simulink model "LAB11_sim_1"  (R2022b)
settings: Solver=VariableStepAuto  StartTime=0.0  StopTime=czas_symulacji  MaxStep=0.1  RelTol=1e-3
values from neighbouring files (symbols this model uses):
  Cvp = cp*rop*Vp    (= 14400)    [LAB11_1.m]
  Cvw = cp*rop*Vw    (= 96000)    [LAB11_1.m]
  drugi_step_time = 3000    [LAB11_1.m]
  dTp = 2    [LAB11_1.m]
  dTp2 = 10    [LAB11_1.m]
  dTzew = 0    [LAB11_1.m]
  Kb = 500    [LAB11_1.m]
  Kcp = (a*QgN)*(TwewN-TpN)/((TpN-TzewN)*(TwewN-TzewN+a*(TwewN-TpN)))    (= 23.2558139535)    [LAB11_1.m]
  Kcw = (QgN)/(TwewN-TzewN+a*TwewN-a*TpN)    (= 232.558139535)    [LAB11_1.m]
  Kcwp = (a*QgN)/(TwewN-TzewN+a*TwewN-a*TpN)    (= 69.7674418605)    [LAB11_1.m]
  lower_limit = 0    [LAB11_1.m]
  spadekTp = -10    [LAB11_1.m]
  t0 = 1000    [LAB11_1.m]
  Tp0 = (Kcp*Tzew0*(Kcw+Kcwp)+Kcwp*(Qg0+Kcw*Tzew0))/(Kcw*Kcwp+Kcw*Kcp+Kcwp*Kcp)    (= 17)    [LAB11_1.m]
  Twew0 = (Qg0+Kcw*Tzew0+a*Kcw*Tp0)/(Kcw+Kcwp)    (= 27)    [LAB11_1.m]
  Tzew0 = TzewN+7    (= -13)    [LAB11_1.m]
  upper_limit = 11500    [LAB11_1.m]
libraries: slpidlib x6
settings Model: Creator=maciejrudy  LastModifiedBy=Dawkin
settings SolverCC: AlgebraicLoopSolver=TrustRegion
settings DataIOCC: ReturnWorkspaceOutputs=off
settings DebuggingCC: UnconnectedInputMsg=warning  UnconnectedOutputMsg=warning  UnconnectedLineMsg=warning  SFMachineParentedDataDiag=warning
settings ModelReferenceCC: EnableRefExpFcnMdlSchedulingChecks=on
settings RTWCC: DLArmComputeVersion=19.05

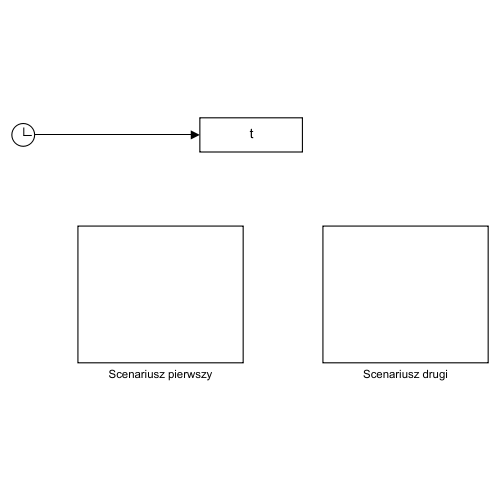
[thumbnail: Simulink's stored preview of the top-level diagram]
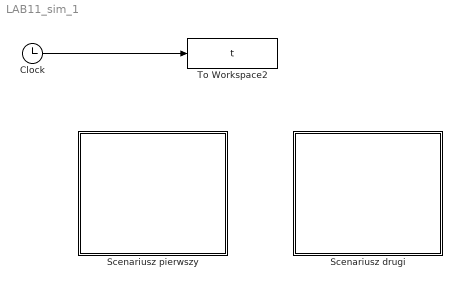
== system LAB11_sim_1 ==
  Clock : Clock
  Scenariusz drugi : Subsystem
  Scenariusz pierwszy : Subsystem
  To Workspace2 : ToWorkspace  VariableName=t  SaveFormat=Timeseries  SampleTime=-1
  wires:
  Clock/1 -> To Workspace2/1

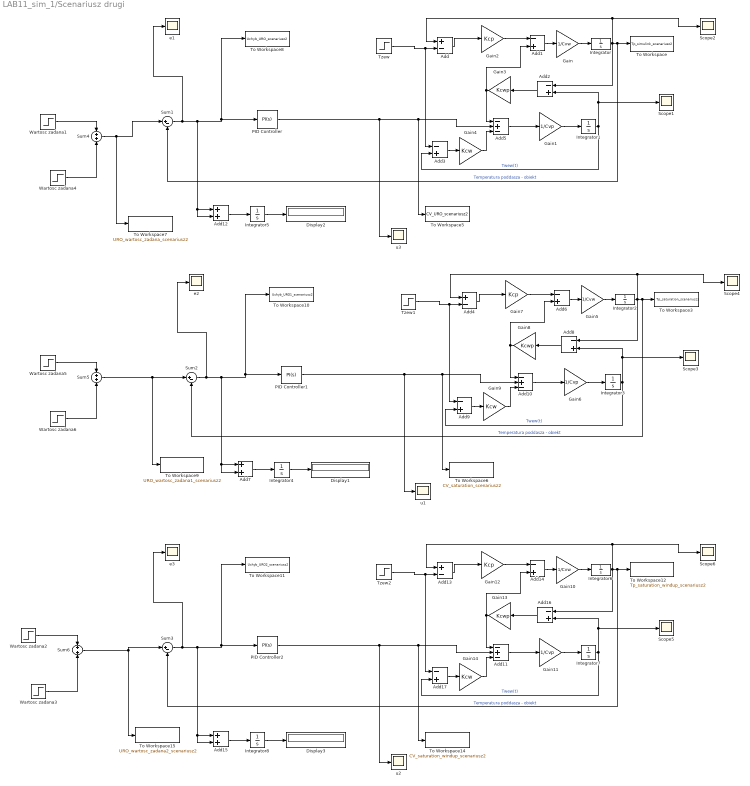
== system LAB11_sim_1/Scenariusz drugi ==
  Add : Sum  Inputs=+-
  Add{1..3,6,8..9,14,16..17} (9 alike) : Sum  Inputs=-+
  Add10 : Sum  Inputs=-+-
  Add11 : Sum  Inputs=-+-
  Add12 : Sum
  Add13 : Sum  Inputs=+-
  Add15 : Sum
  Add4 : Sum  Inputs=+-
  Add5 : Sum  Inputs=-+-
  Add7 : Sum
  Display1 : Display
  Display2 : Display
  Display3 : Display
  Gain : Gain  Gain=1/Cvw
  Gain1 : Gain  Gain=1/Cvp
  Gain10 : Gain  Gain=1/Cvw
  Gain11 : Gain  Gain=1/Cvp
  Gain12 : Gain  Gain=Kcp
  Gain13 : Gain  Gain=Kcwp
  Gain14 : Gain  Gain=Kcw
  Gain2 : Gain  Gain=Kcp
  Gain3 : Gain  Gain=Kcwp
  Gain4 : Gain  Gain=Kcw
  Gain5 : Gain  Gain=1/Cvw
  Gain6 : Gain  Gain=1/Cvp
  Gain7 : Gain  Gain=Kcp
  Gain8 : Gain  Gain=Kcwp
  Gain9 : Gain  Gain=Kcw
  Integrator : Integrator  InitialCondition=Tp0
  Integrator1 : Integrator  InitialCondition=Twew0
  Integrator2 : Integrator  InitialCondition=Tp0
  Integrator3 : Integrator  InitialCondition=Twew0
  Integrator4 : Integrator
  Integrator5 : Integrator
  Integrator6 : Integrator  InitialCondition=Tp0
  Integrator7 : Integrator  InitialCondition=Twew0
  Integrator8 : Integrator
  PID Controller : slpidlib/PID Controller  Controller=PI  Form=Parallel  TimeDomain=Continuous-time  UseExternalTs=off  SampleTime=-1  IntegratorMethod=Forward Euler  FilterMethod=Forward Euler  ControllerParametersSource=internal  P=2386.66771221404  I=38.2166019284268  UseKiTs=off  D=0  N=100  UseFilter=on  TunerSelectOption=Transfer Function Based (PID Tuner App)  InitialConditionSource=internal  InitialConditionForIntegrator=Qg0  InitialConditionForFilter=0  DifferentiatorICPrevScaledInput=0  ExternalReset=none  TrackingMode=off  Kt=1  LimitOutput=off  SatLimitsSource=internal  UpperSaturationLimit=upper_limit  LowerSaturationLimit=lower_limit  LinearizeAsGain=on  AntiWindupMode=back-calculation  Kb=Kb  LimitIntegrator=off  UpperIntegratorSaturationLimit=inf  LowerIntegratorSaturationLimit=-inf  POutMin=[]  POutMax=[]  IOutMin=[]  IOutMax=[]  DOutMin=[]  DOutMax=[]  NOutMin=[]  NOutMax=[]  SumOutMin=[]  SumOutMax=[]  SaturationOutMin=[]  SaturationOutMax=[]  PParamMin=[]  PParamMax=[]  IParamMin=[]  IParamMax=[]  DParamMin=[]  DParamMax=[]  NParamMin=[]  NParamMax=[]  KbParamMin=[]  KbParamMax=[]  KtParamMin=[]  KtParamMax=[]  KbOutMin=[]  KbOutMax=[]  KtOutMin=[]  KtOutMax=[]  IntegratorOutMin=[]  IntegratorOutMax=[]  FilterOutMin=[]  FilterOutMax=[]  SumI1OutMin=[]  SumI1OutMax=[]  SumI2OutMin=[]  SumI2OutMax=[]  SumI3OutMin=[]  SumI3OutMax=[]  SumI4OutMin=[]  SumI4OutMax=[]  SumDOutMin=[]  SumDOutMax=[]  DifferentiatorOutMin=[]  DifferentiatorOutMax=[]  FilterDiffOutCoefMin=[]  FilterDiffOutCoefMax=[]  ReciprocalOutMin=[]  ReciprocalOutMax=[]  SumDenOutMin=[]  SumDenOutMax=[]  SumNumOutMin=[]  SumNumOutMax=[]  DivideOutMin=[]  DivideOutMax=[]  UdiffTsProdOutMin=[]  UdiffTsProdOutMax=[]  NTsProdOutMin=[]  NTsProdOutMax=[]  UintegralTsProdOutMin=[]  UintegralTsProdOutMax=[]  UngainTsProdOutMin=[]  UngainTsProdOutMax=[]  ClampingZeroOutDataTypeStr=Inherit: Inherit via back propagation  ClampingZeroOutMin=[]  ClampingZeroOutMax=[]  FilterDenConstantOutDataTypeStr=Inherit: Inherit via back propagation  FilterDenConstantOutMin=[]  FilterDenConstantOutMax=[]  PCopyOutDataTypeStr=Inherit: Inherit via back propagation  PCopyOutMin=[]  PCopyOutMax=[]  NCopyOutDataTypeStr=Inherit: Inherit via back propagation  NCopyOutMin=[]  NCopyOutMax=[]  IntegratorContinuousStateAttributes=''  IntegratorStateMustResolveToSignalObject=off  IntegratorRTWStateStorageClass=Auto  FilterContinuousStateAttributes=''  FilterStateMustResolveToSignalObject=off  FilterRTWStateStorageClass=Auto  ParallelPVariant=InternalParameters  IdealPVariant=Disabled  IVariant=InternalParameters  DVariant=Disabled  IntegratorVariant=Continuous  SatVariant=Disabled  AWVariant=Passthrough  PCopyVariant=Disabled  TRVariant=Disabled  FdbkBlocksVariant=Forward  IdealPFdbkVariant=Disabled  SatFdbkVariant=Disabled  DerivativeFilterVariant=Disabled  NVariant=Disabled  NCopyVariant=Disabled_SignalSpec  FilterICVariant=Disabled  IntegratorICVariant=InternalICs  ExternalResetVariant=Disabled  TRSumVariant=Passthrough  SumFdbkVariant=Disabled  SumVariant=Sum_PI  TsampFilterVariant=InternalTs  TsampNgainVariant=Passthrough  TsampIntegralVariant=Passthrough  ExternalSaturationOutDataTypeStr=Inherit: Same as second input
  PID Controller1 : slpidlib/PID Controller  Controller=PI  Form=Parallel  TimeDomain=Continuous-time  UseExternalTs=off  SampleTime=-1  IntegratorMethod=Forward Euler  FilterMethod=Forward Euler  ControllerParametersSource=internal  P=2386.66771221404  I=38.2166019284268  UseKiTs=off  D=0  N=100  UseFilter=on  TunerSelectOption=Transfer Function Based (PID Tuner App)  InitialConditionSource=internal  InitialConditionForIntegrator=Qg0  InitialConditionForFilter=0  DifferentiatorICPrevScaledInput=0  ExternalReset=none  TrackingMode=off  Kt=1  LimitOutput=on  SatLimitsSource=internal  UpperSaturationLimit=upper_limit  LowerSaturationLimit=lower_limit  LinearizeAsGain=on  AntiWindupMode=none  Kb=Kb  LimitIntegrator=off  UpperIntegratorSaturationLimit=inf  LowerIntegratorSaturationLimit=-inf  POutMin=[]  POutMax=[]  IOutMin=[]  IOutMax=[]  DOutMin=[]  DOutMax=[]  NOutMin=[]  NOutMax=[]  SumOutMin=[]  SumOutMax=[]  SaturationOutMin=[]  SaturationOutMax=[]  PParamMin=[]  PParamMax=[]  IParamMin=[]  IParamMax=[]  DParamMin=[]  DParamMax=[]  NParamMin=[]  NParamMax=[]  KbParamMin=[]  KbParamMax=[]  KtParamMin=[]  KtParamMax=[]  KbOutMin=[]  KbOutMax=[]  KtOutMin=[]  KtOutMax=[]  IntegratorOutMin=[]  IntegratorOutMax=[]  FilterOutMin=[]  FilterOutMax=[]  SumI1OutMin=[]  SumI1OutMax=[]  SumI2OutMin=[]  SumI2OutMax=[]  SumI3OutMin=[]  SumI3OutMax=[]  SumI4OutMin=[]  SumI4OutMax=[]  SumDOutMin=[]  SumDOutMax=[]  DifferentiatorOutMin=[]  DifferentiatorOutMax=[]  FilterDiffOutCoefMin=[]  FilterDiffOutCoefMax=[]  ReciprocalOutMin=[]  ReciprocalOutMax=[]  SumDenOutMin=[]  SumDenOutMax=[]  SumNumOutMin=[]  SumNumOutMax=[]  DivideOutMin=[]  DivideOutMax=[]  UdiffTsProdOutMin=[]  UdiffTsProdOutMax=[]  NTsProdOutMin=[]  NTsProdOutMax=[]  UintegralTsProdOutMin=[]  UintegralTsProdOutMax=[]  UngainTsProdOutMin=[]  UngainTsProdOutMax=[]  ClampingZeroOutDataTypeStr=Inherit: Inherit via back propagation  ClampingZeroOutMin=[]  ClampingZeroOutMax=[]  FilterDenConstantOutDataTypeStr=Inherit: Inherit via back propagation  FilterDenConstantOutMin=[]  FilterDenConstantOutMax=[]  PCopyOutDataTypeStr=Inherit: Inherit via back propagation  PCopyOutMin=[]  PCopyOutMax=[]  NCopyOutDataTypeStr=Inherit: Inherit via back propagation  NCopyOutMin=[]  NCopyOutMax=[]  IntegratorContinuousStateAttributes=''  IntegratorStateMustResolveToSignalObject=off  IntegratorRTWStateStorageClass=Auto  FilterContinuousStateAttributes=''  FilterStateMustResolveToSignalObject=off  FilterRTWStateStorageClass=Auto  ParallelPVariant=InternalParameters  IdealPVariant=Disabled  IVariant=InternalParameters  DVariant=Disabled  IntegratorVariant=Continuous  SatVariant=Enabled  AWVariant=Passthrough  PCopyVariant=Disabled  TRVariant=Disabled  FdbkBlocksVariant=Forward  IdealPFdbkVariant=Disabled  SatFdbkVariant=Disabled  DerivativeFilterVariant=Disabled  NVariant=Disabled  NCopyVariant=Disabled_SignalSpec  FilterICVariant=Disabled  IntegratorICVariant=InternalICs  ExternalResetVariant=Disabled  TRSumVariant=Passthrough  SumFdbkVariant=Disabled  SumVariant=Sum_PI  TsampFilterVariant=InternalTs  TsampNgainVariant=Passthrough  TsampIntegralVariant=Passthrough  ExternalSaturationOutDataTypeStr=Inherit: Same as second input
  PID Controller2 : slpidlib/PID Controller  Controller=PI  Form=Parallel  TimeDomain=Continuous-time  UseExternalTs=off  SampleTime=-1  IntegratorMethod=Forward Euler  FilterMethod=Forward Euler  ControllerParametersSource=internal  P=2386.66771221404  I=38.2166019284268  UseKiTs=off  D=0  N=100  UseFilter=on  TunerSelectOption=Transfer Function Based (PID Tuner App)  InitialConditionSource=internal  InitialConditionForIntegrator=Qg0  InitialConditionForFilter=0  DifferentiatorICPrevScaledInput=0  ExternalReset=none  TrackingMode=off  Kt=1  LimitOutput=on  SatLimitsSource=internal  UpperSaturationLimit=upper_limit  LowerSaturationLimit=lower_limit  LinearizeAsGain=on  AntiWindupMode=back-calculation  Kb=Kb  LimitIntegrator=off  UpperIntegratorSaturationLimit=inf  LowerIntegratorSaturationLimit=-inf  POutMin=[]  POutMax=[]  IOutMin=[]  IOutMax=[]  DOutMin=[]  DOutMax=[]  NOutMin=[]  NOutMax=[]  SumOutMin=[]  SumOutMax=[]  SaturationOutMin=[]  SaturationOutMax=[]  PParamMin=[]  PParamMax=[]  IParamMin=[]  IParamMax=[]  DParamMin=[]  DParamMax=[]  NParamMin=[]  NParamMax=[]  KbParamMin=[]  KbParamMax=[]  KtParamMin=[]  KtParamMax=[]  KbOutMin=[]  KbOutMax=[]  KtOutMin=[]  KtOutMax=[]  IntegratorOutMin=[]  IntegratorOutMax=[]  FilterOutMin=[]  FilterOutMax=[]  SumI1OutMin=[]  SumI1OutMax=[]  SumI2OutMin=[]  SumI2OutMax=[]  SumI3OutMin=[]  SumI3OutMax=[]  SumI4OutMin=[]  SumI4OutMax=[]  SumDOutMin=[]  SumDOutMax=[]  DifferentiatorOutMin=[]  DifferentiatorOutMax=[]  FilterDiffOutCoefMin=[]  FilterDiffOutCoefMax=[]  ReciprocalOutMin=[]  ReciprocalOutMax=[]  SumDenOutMin=[]  SumDenOutMax=[]  SumNumOutMin=[]  SumNumOutMax=[]  DivideOutMin=[]  DivideOutMax=[]  UdiffTsProdOutMin=[]  UdiffTsProdOutMax=[]  NTsProdOutMin=[]  NTsProdOutMax=[]  UintegralTsProdOutMin=[]  UintegralTsProdOutMax=[]  UngainTsProdOutMin=[]  UngainTsProdOutMax=[]  ClampingZeroOutDataTypeStr=Inherit: Inherit via back propagation  ClampingZeroOutMin=[]  ClampingZeroOutMax=[]  FilterDenConstantOutDataTypeStr=Inherit: Inherit via back propagation  FilterDenConstantOutMin=[]  FilterDenConstantOutMax=[]  PCopyOutDataTypeStr=Inherit: Inherit via back propagation  PCopyOutMin=[]  PCopyOutMax=[]  NCopyOutDataTypeStr=Inherit: Inherit via back propagation  NCopyOutMin=[]  NCopyOutMax=[]  IntegratorContinuousStateAttributes=''  IntegratorStateMustResolveToSignalObject=off  IntegratorRTWStateStorageClass=Auto  FilterContinuousStateAttributes=''  FilterStateMustResolveToSignalObject=off  FilterRTWStateStorageClass=Auto  ParallelPVariant=InternalParameters  IdealPVariant=Disabled  IVariant=InternalParameters  DVariant=Disabled  IntegratorVariant=Continuous  SatVariant=Enabled  AWVariant=BackCalculation  PCopyVariant=Disabled  TRVariant=Disabled  FdbkBlocksVariant=Forward  IdealPFdbkVariant=Disabled  SatFdbkVariant=Disabled  DerivativeFilterVariant=Disabled  NVariant=Disabled  NCopyVariant=Disabled_SignalSpec  FilterICVariant=Disabled  IntegratorICVariant=InternalICs  ExternalResetVariant=Disabled  TRSumVariant=Passthrough  SumFdbkVariant=Disabled  SumVariant=Sum_PI  TsampFilterVariant=InternalTs  TsampNgainVariant=Passthrough  TsampIntegralVariant=Passthrough  ExternalSaturationOutDataTypeStr=Inherit: Same as second input
  Scope{1..6} (6 alike) : Scope
  Sum1 : Sum  Inputs=|+-
  Sum2 : Sum  Inputs=|+-
  Sum3 : Sum  Inputs=|+-
  Sum4 : Sum
  Sum5 : Sum
  Sum6 : Sum
  To Workspace : ToWorkspace  VariableName=Tp_simulink_scenariusz2  SampleTime=-1
  To Workspace10 : ToWorkspace  VariableName=Uchyb_URO1_scenariusz2  SampleTime=-1
  To Workspace11 : ToWorkspace  VariableName=Uchyb_URO2_scenariusz2  SampleTime=-1
  To Workspace12 : ToWorkspace  VariableName=Tp_saturation_windup_scenariusz2  SampleTime=-1
  To Workspace14 : ToWorkspace  VariableName=CV_saturation_windup_scenariusz2  SampleTime=-1
  To Workspace15 : ToWorkspace  VariableName=URO_wartosc_zadana2_scenariusz2  SampleTime=-1
  To Workspace3 : ToWorkspace  VariableName=Tp_saturation_scenariusz2  SampleTime=-1
  To Workspace5 : ToWorkspace  VariableName=CV_URO_scenariusz2  SampleTime=-1
  To Workspace6 : ToWorkspace  VariableName=CV_saturation_scenariusz2  SampleTime=-1
  To Workspace7 : ToWorkspace  VariableName=URO_wartosc_zadana_scenariusz2  SampleTime=-1
  To Workspace8 : ToWorkspace  VariableName=Uchyb_URO_scenariusz2  SampleTime=-1
  To Workspace9 : ToWorkspace  VariableName=URO_wartosc_zadana1_scenariusz2  SampleTime=-1
  Tzew : Step  Time=t0  Before=Tzew0  After=Tzew0+dTzew  SampleTime=0
  Tzew1 : Step  Time=t0  Before=Tzew0  After=Tzew0+dTzew  SampleTime=0
  Tzew2 : Step  Time=t0  Before=Tzew0  After=Tzew0+dTzew  SampleTime=0
  Wartosc zadana1 : Step  Time=t0  Before=Tp0  After=Tp0+dTp2  SampleTime=0
  Wartosc zadana2 : Step  Time=t0  Before=Tp0  After=Tp0+dTp2  SampleTime=0
  Wartosc zadana3 : Step  Time=drugi_step_time  After=spadekTp  SampleTime=0
  Wartosc zadana4 : Step  Time=drugi_step_time  After=spadekTp  SampleTime=0
  Wartosc zadana5 : Step  Time=t0  Before=Tp0  After=Tp0+dTp2  SampleTime=0
  Wartosc zadana6 : Step  Time=drugi_step_time  After=spadekTp  SampleTime=0
  e1 : Scope
  e2 : Scope
  e3 : Scope
  u1 : Scope
  u2 : Scope
  u3 : Scope
  wires:
  Gain12/1 -> Add14/1
  Gain11/1 -> Integrator7/1
  Integrator6/1 -> Add16/1, To Workspace12/1, Sum3/2, Scope6/1, Add13/1  "Temperatura poddasza - obiekt"
  Add17/1 -> Gain14/1
  Gain4/1 -> Add5/3
  Add5/1 -> Gain1/1
  Gain14/1 -> Add11/3
  Gain/1 -> Integrator/1
  Tzew2/1 -> Add17/1, Add13/2
  Add/1 -> Gain2/1
  Add15/1 -> Integrator8/1
  Add8/1 -> Gain8/1
  Add10/1 -> Gain6/1
  PID Controller/1 -> To Workspace5/1, Add5/2, u3/1
  Add12/1 -> Integrator5/1
  Gain6/1 -> Integrator3/1
  Add7/1 -> Integrator4/1
  Add2/1 -> Gain3/1
  Gain3/1 -> Add5/1, Add1/2
  Add9/1 -> Gain9/1
  PID Controller2/1 -> To Workspace14/1, Add11/2, u2/1
  Add11/1 -> Gain11/1
  Gain13/1 -> Add11/1, Add14/2
  Tzew/1 -> Add3/1, Add/2
  Integrator8/1 -> Display3/1
  Gain1/1 -> Integrator1/1
  Add16/1 -> Gain13/1
  Integrator7/1 -> Add17/2, Add16/2, Scope5/1  "Twew(t)"
  Add13/1 -> Gain12/1
  Integrator/1 -> Add2/1, To Workspace/1, Sum1/2, Scope2/1, Add/1  "Temperatura poddasza - obiekt"
  Gain9/1 -> Add10/3
  Integrator5/1 -> Display2/1
  Sum6/1 -> Sum3/1, To Workspace15/1
  Gain5/1 -> Integrator2/1
  Tzew1/1 -> Add9/1, Add4/2
  Add14/1 -> Gain10/1
  Integrator4/1 -> Display1/1
  Sum5/1 -> To Workspace9/1, Sum2/1
  Integrator3/1 -> Add9/2, Add8/2, Scope3/1  "Twew(t)"
  Add6/1 -> Gain5/1
  Add3/1 -> Gain4/1
  Gain2/1 -> Add1/1
  Add1/1 -> Gain/1
  Sum2/1 -> e2/1, PID Controller1/1, To Workspace10/1, Add7/2, Add7/1
  PID Controller1/1 -> To Workspace6/1, Add10/2, u1/1
  Sum1/1 -> e1/1, PID Controller/1, To Workspace8/1, Add12/2, Add12/1
  Gain7/1 -> Add6/1
  Gain8/1 -> Add10/1, Add6/2
  Integrator1/1 -> Add3/2, Add2/2, Scope1/1  "Twew(t)"
  Sum3/1 -> e3/1, PID Controller2/1, To Workspace11/1, Add15/2, Add15/1
  Gain10/1 -> Integrator6/1
  Integrator2/1 -> Add8/1, To Workspace3/1, Sum2/2, Scope4/1, Add4/1  "Temperatura poddasza - obiekt"
  Add4/1 -> Gain7/1
  Wartosc zadana4/1 -> Sum4/2
  Wartosc zadana1/1 -> Sum4/1
  Sum4/1 -> Sum1/1, To Workspace7/1
  Wartosc zadana6/1 -> Sum5/2
  Wartosc zadana5/1 -> Sum5/1
  Wartosc zadana3/1 -> Sum6/2
  Wartosc zadana2/1 -> Sum6/1

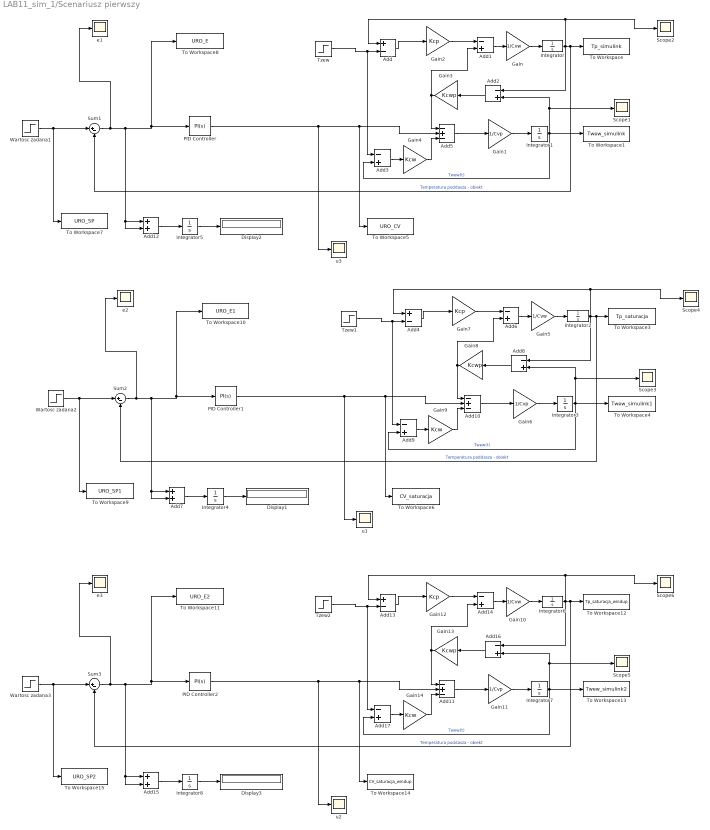
== system LAB11_sim_1/Scenariusz pierwszy ==
  Add : Sum  Inputs=+-
  Add{1..3,6,8..9,14,16..17} (9 alike) : Sum  Inputs=-+
  Add10 : Sum  Inputs=-+-
  Add11 : Sum  Inputs=-+-
  Add12 : Sum
  Add13 : Sum  Inputs=+-
  Add15 : Sum
  Add4 : Sum  Inputs=+-
  Add5 : Sum  Inputs=-+-
  Add7 : Sum
  Display1 : Display
  Display2 : Display
  Display3 : Display
  Gain : Gain  Gain=1/Cvw
  Gain1 : Gain  Gain=1/Cvp
  Gain10 : Gain  Gain=1/Cvw
  Gain11 : Gain  Gain=1/Cvp
  Gain12 : Gain  Gain=Kcp
  Gain13 : Gain  Gain=Kcwp
  Gain14 : Gain  Gain=Kcw
  Gain2 : Gain  Gain=Kcp
  Gain3 : Gain  Gain=Kcwp
  Gain4 : Gain  Gain=Kcw
  Gain5 : Gain  Gain=1/Cvw
  Gain6 : Gain  Gain=1/Cvp
  Gain7 : Gain  Gain=Kcp
  Gain8 : Gain  Gain=Kcwp
  Gain9 : Gain  Gain=Kcw
  Integrator : Integrator  InitialCondition=Tp0
  Integrator1 : Integrator  InitialCondition=Twew0
  Integrator2 : Integrator  InitialCondition=Tp0
  Integrator3 : Integrator  InitialCondition=Twew0
  Integrator4 : Integrator
  Integrator5 : Integrator
  Integrator6 : Integrator  InitialCondition=Tp0
  Integrator7 : Integrator  InitialCondition=Twew0
  Integrator8 : Integrator
  PID Controller : slpidlib/PID Controller  Controller=PI  Form=Parallel  TimeDomain=Continuous-time  UseExternalTs=off  SampleTime=-1  IntegratorMethod=Forward Euler  FilterMethod=Forward Euler  ControllerParametersSource=internal  P=2386.66771221404  I=38.2166019284268  UseKiTs=off  D=0  N=100  UseFilter=on  TunerSelectOption=Transfer Function Based (PID Tuner App)  InitialConditionSource=internal  InitialConditionForIntegrator=Qg0  InitialConditionForFilter=0  DifferentiatorICPrevScaledInput=0  ExternalReset=none  TrackingMode=off  Kt=1  LimitOutput=off  SatLimitsSource=internal  UpperSaturationLimit=upper_limit  LowerSaturationLimit=lower_limit  LinearizeAsGain=on  AntiWindupMode=back-calculation  Kb=Kb  LimitIntegrator=off  UpperIntegratorSaturationLimit=inf  LowerIntegratorSaturationLimit=-inf  POutMin=[]  POutMax=[]  IOutMin=[]  IOutMax=[]  DOutMin=[]  DOutMax=[]  NOutMin=[]  NOutMax=[]  SumOutMin=[]  SumOutMax=[]  SaturationOutMin=[]  SaturationOutMax=[]  PParamMin=[]  PParamMax=[]  IParamMin=[]  IParamMax=[]  DParamMin=[]  DParamMax=[]  NParamMin=[]  NParamMax=[]  KbParamMin=[]  KbParamMax=[]  KtParamMin=[]  KtParamMax=[]  KbOutMin=[]  KbOutMax=[]  KtOutMin=[]  KtOutMax=[]  IntegratorOutMin=[]  IntegratorOutMax=[]  FilterOutMin=[]  FilterOutMax=[]  SumI1OutMin=[]  SumI1OutMax=[]  SumI2OutMin=[]  SumI2OutMax=[]  SumI3OutMin=[]  SumI3OutMax=[]  SumI4OutMin=[]  SumI4OutMax=[]  SumDOutMin=[]  SumDOutMax=[]  DifferentiatorOutMin=[]  DifferentiatorOutMax=[]  FilterDiffOutCoefMin=[]  FilterDiffOutCoefMax=[]  ReciprocalOutMin=[]  ReciprocalOutMax=[]  SumDenOutMin=[]  SumDenOutMax=[]  SumNumOutMin=[]  SumNumOutMax=[]  DivideOutMin=[]  DivideOutMax=[]  UdiffTsProdOutMin=[]  UdiffTsProdOutMax=[]  NTsProdOutMin=[]  NTsProdOutMax=[]  UintegralTsProdOutMin=[]  UintegralTsProdOutMax=[]  UngainTsProdOutMin=[]  UngainTsProdOutMax=[]  ClampingZeroOutDataTypeStr=Inherit: Inherit via back propagation  ClampingZeroOutMin=[]  ClampingZeroOutMax=[]  FilterDenConstantOutDataTypeStr=Inherit: Inherit via back propagation  FilterDenConstantOutMin=[]  FilterDenConstantOutMax=[]  PCopyOutDataTypeStr=Inherit: Inherit via back propagation  PCopyOutMin=[]  PCopyOutMax=[]  NCopyOutDataTypeStr=Inherit: Inherit via back propagation  NCopyOutMin=[]  NCopyOutMax=[]  IntegratorContinuousStateAttributes=''  IntegratorStateMustResolveToSignalObject=off  IntegratorRTWStateStorageClass=Auto  FilterContinuousStateAttributes=''  FilterStateMustResolveToSignalObject=off  FilterRTWStateStorageClass=Auto  ParallelPVariant=InternalParameters  IdealPVariant=Disabled  IVariant=InternalParameters  DVariant=Disabled  IntegratorVariant=Continuous  SatVariant=Disabled  AWVariant=Passthrough  PCopyVariant=Disabled  TRVariant=Disabled  FdbkBlocksVariant=Forward  IdealPFdbkVariant=Disabled  SatFdbkVariant=Disabled  DerivativeFilterVariant=Disabled  NVariant=Disabled  NCopyVariant=Disabled_SignalSpec  FilterICVariant=Disabled  IntegratorICVariant=InternalICs  ExternalResetVariant=Disabled  TRSumVariant=Passthrough  SumFdbkVariant=Disabled  SumVariant=Sum_PI  TsampFilterVariant=InternalTs  TsampNgainVariant=Passthrough  TsampIntegralVariant=Passthrough  ExternalSaturationOutDataTypeStr=Inherit: Same as second input
  PID Controller1 : slpidlib/PID Controller  Controller=PI  Form=Parallel  TimeDomain=Continuous-time  UseExternalTs=off  SampleTime=-1  IntegratorMethod=Forward Euler  FilterMethod=Forward Euler  ControllerParametersSource=internal  P=2386.66771221404  I=38.2166019284268  UseKiTs=off  D=0  N=100  UseFilter=on  TunerSelectOption=Transfer Function Based (PID Tuner App)  InitialConditionSource=internal  InitialConditionForIntegrator=Qg0  InitialConditionForFilter=0  DifferentiatorICPrevScaledInput=0  ExternalReset=none  TrackingMode=off  Kt=1  LimitOutput=on  SatLimitsSource=internal  UpperSaturationLimit=upper_limit  LowerSaturationLimit=lower_limit  LinearizeAsGain=on  AntiWindupMode=none  Kb=Kb  LimitIntegrator=off  UpperIntegratorSaturationLimit=inf  LowerIntegratorSaturationLimit=-inf  POutMin=[]  POutMax=[]  IOutMin=[]  IOutMax=[]  DOutMin=[]  DOutMax=[]  NOutMin=[]  NOutMax=[]  SumOutMin=[]  SumOutMax=[]  SaturationOutMin=[]  SaturationOutMax=[]  PParamMin=[]  PParamMax=[]  IParamMin=[]  IParamMax=[]  DParamMin=[]  DParamMax=[]  NParamMin=[]  NParamMax=[]  KbParamMin=[]  KbParamMax=[]  KtParamMin=[]  KtParamMax=[]  KbOutMin=[]  KbOutMax=[]  KtOutMin=[]  KtOutMax=[]  IntegratorOutMin=[]  IntegratorOutMax=[]  FilterOutMin=[]  FilterOutMax=[]  SumI1OutMin=[]  SumI1OutMax=[]  SumI2OutMin=[]  SumI2OutMax=[]  SumI3OutMin=[]  SumI3OutMax=[]  SumI4OutMin=[]  SumI4OutMax=[]  SumDOutMin=[]  SumDOutMax=[]  DifferentiatorOutMin=[]  DifferentiatorOutMax=[]  FilterDiffOutCoefMin=[]  FilterDiffOutCoefMax=[]  ReciprocalOutMin=[]  ReciprocalOutMax=[]  SumDenOutMin=[]  SumDenOutMax=[]  SumNumOutMin=[]  SumNumOutMax=[]  DivideOutMin=[]  DivideOutMax=[]  UdiffTsProdOutMin=[]  UdiffTsProdOutMax=[]  NTsProdOutMin=[]  NTsProdOutMax=[]  UintegralTsProdOutMin=[]  UintegralTsProdOutMax=[]  UngainTsProdOutMin=[]  UngainTsProdOutMax=[]  ClampingZeroOutDataTypeStr=Inherit: Inherit via back propagation  ClampingZeroOutMin=[]  ClampingZeroOutMax=[]  FilterDenConstantOutDataTypeStr=Inherit: Inherit via back propagation  FilterDenConstantOutMin=[]  FilterDenConstantOutMax=[]  PCopyOutDataTypeStr=Inherit: Inherit via back propagation  PCopyOutMin=[]  PCopyOutMax=[]  NCopyOutDataTypeStr=Inherit: Inherit via back propagation  NCopyOutMin=[]  NCopyOutMax=[]  IntegratorContinuousStateAttributes=''  IntegratorStateMustResolveToSignalObject=off  IntegratorRTWStateStorageClass=Auto  FilterContinuousStateAttributes=''  FilterStateMustResolveToSignalObject=off  FilterRTWStateStorageClass=Auto  ParallelPVariant=InternalParameters  IdealPVariant=Disabled  IVariant=InternalParameters  DVariant=Disabled  IntegratorVariant=Continuous  SatVariant=Enabled  AWVariant=Passthrough  PCopyVariant=Disabled  TRVariant=Disabled  FdbkBlocksVariant=Forward  IdealPFdbkVariant=Disabled  SatFdbkVariant=Disabled  DerivativeFilterVariant=Disabled  NVariant=Disabled  NCopyVariant=Disabled_SignalSpec  FilterICVariant=Disabled  IntegratorICVariant=InternalICs  ExternalResetVariant=Disabled  TRSumVariant=Passthrough  SumFdbkVariant=Disabled  SumVariant=Sum_PI  TsampFilterVariant=InternalTs  TsampNgainVariant=Passthrough  TsampIntegralVariant=Passthrough  ExternalSaturationOutDataTypeStr=Inherit: Same as second input
  PID Controller2 : slpidlib/PID Controller  Controller=PI  Form=Parallel  TimeDomain=Continuous-time  UseExternalTs=off  SampleTime=-1  IntegratorMethod=Forward Euler  FilterMethod=Forward Euler  ControllerParametersSource=internal  P=2386.66771221404  I=38.2166019284268  UseKiTs=off  D=0  N=100  UseFilter=on  TunerSelectOption=Transfer Function Based (PID Tuner App)  InitialConditionSource=internal  InitialConditionForIntegrator=Qg0  InitialConditionForFilter=0  DifferentiatorICPrevScaledInput=0  ExternalReset=none  TrackingMode=off  Kt=1  LimitOutput=on  SatLimitsSource=internal  UpperSaturationLimit=upper_limit  LowerSaturationLimit=lower_limit  LinearizeAsGain=on  AntiWindupMode=back-calculation  Kb=Kb  LimitIntegrator=off  UpperIntegratorSaturationLimit=inf  LowerIntegratorSaturationLimit=-inf  POutMin=[]  POutMax=[]  IOutMin=[]  IOutMax=[]  DOutMin=[]  DOutMax=[]  NOutMin=[]  NOutMax=[]  SumOutMin=[]  SumOutMax=[]  SaturationOutMin=[]  SaturationOutMax=[]  PParamMin=[]  PParamMax=[]  IParamMin=[]  IParamMax=[]  DParamMin=[]  DParamMax=[]  NParamMin=[]  NParamMax=[]  KbParamMin=[]  KbParamMax=[]  KtParamMin=[]  KtParamMax=[]  KbOutMin=[]  KbOutMax=[]  KtOutMin=[]  KtOutMax=[]  IntegratorOutMin=[]  IntegratorOutMax=[]  FilterOutMin=[]  FilterOutMax=[]  SumI1OutMin=[]  SumI1OutMax=[]  SumI2OutMin=[]  SumI2OutMax=[]  SumI3OutMin=[]  SumI3OutMax=[]  SumI4OutMin=[]  SumI4OutMax=[]  SumDOutMin=[]  SumDOutMax=[]  DifferentiatorOutMin=[]  DifferentiatorOutMax=[]  FilterDiffOutCoefMin=[]  FilterDiffOutCoefMax=[]  ReciprocalOutMin=[]  ReciprocalOutMax=[]  SumDenOutMin=[]  SumDenOutMax=[]  SumNumOutMin=[]  SumNumOutMax=[]  DivideOutMin=[]  DivideOutMax=[]  UdiffTsProdOutMin=[]  UdiffTsProdOutMax=[]  NTsProdOutMin=[]  NTsProdOutMax=[]  UintegralTsProdOutMin=[]  UintegralTsProdOutMax=[]  UngainTsProdOutMin=[]  UngainTsProdOutMax=[]  ClampingZeroOutDataTypeStr=Inherit: Inherit via back propagation  ClampingZeroOutMin=[]  ClampingZeroOutMax=[]  FilterDenConstantOutDataTypeStr=Inherit: Inherit via back propagation  FilterDenConstantOutMin=[]  FilterDenConstantOutMax=[]  PCopyOutDataTypeStr=Inherit: Inherit via back propagation  PCopyOutMin=[]  PCopyOutMax=[]  NCopyOutDataTypeStr=Inherit: Inherit via back propagation  NCopyOutMin=[]  NCopyOutMax=[]  IntegratorContinuousStateAttributes=''  IntegratorStateMustResolveToSignalObject=off  IntegratorRTWStateStorageClass=Auto  FilterContinuousStateAttributes=''  FilterStateMustResolveToSignalObject=off  FilterRTWStateStorageClass=Auto  ParallelPVariant=InternalParameters  IdealPVariant=Disabled  IVariant=InternalParameters  DVariant=Disabled  IntegratorVariant=Continuous  SatVariant=Enabled  AWVariant=BackCalculation  PCopyVariant=Disabled  TRVariant=Disabled  FdbkBlocksVariant=Forward  IdealPFdbkVariant=Disabled  SatFdbkVariant=Disabled  DerivativeFilterVariant=Disabled  NVariant=Disabled  NCopyVariant=Disabled_SignalSpec  FilterICVariant=Disabled  IntegratorICVariant=InternalICs  ExternalResetVariant=Disabled  TRSumVariant=Passthrough  SumFdbkVariant=Disabled  SumVariant=Sum_PI  TsampFilterVariant=InternalTs  TsampNgainVariant=Passthrough  TsampIntegralVariant=Passthrough  ExternalSaturationOutDataTypeStr=Inherit: Same as second input
  Scope{1..6} (6 alike) : Scope
  Sum1 : Sum  Inputs=|+-
  Sum2 : Sum  Inputs=|+-
  Sum3 : Sum  Inputs=|+-
  To Workspace : ToWorkspace  VariableName=Tp_simulink  SampleTime=-1
  To Workspace1 : ToWorkspace  VariableName=Twew_simulink  SampleTime=-1
  To Workspace10 : ToWorkspace  VariableName=URO_E1  SampleTime=-1
  To Workspace11 : ToWorkspace  VariableName=URO_E2  SampleTime=-1
  To Workspace12 : ToWorkspace  VariableName=Tp_saturacja_windup  SampleTime=-1
  To Workspace13 : ToWorkspace  VariableName=Twew_simulink2  SampleTime=-1
  To Workspace14 : ToWorkspace  VariableName=CV_saturacja_windup  SampleTime=-1
  To Workspace15 : ToWorkspace  VariableName=URO_SP2  SampleTime=-1
  To Workspace3 : ToWorkspace  VariableName=Tp_saturacja  SampleTime=-1
  To Workspace4 : ToWorkspace  VariableName=Twew_simulink1  SampleTime=-1
  To Workspace5 : ToWorkspace  VariableName=URO_CV  SampleTime=-1
  To Workspace6 : ToWorkspace  VariableName=CV_saturacja  SampleTime=-1
  To Workspace7 : ToWorkspace  VariableName=URO_SP  SampleTime=-1
  To Workspace8 : ToWorkspace  VariableName=URO_E  SampleTime=-1
  To Workspace9 : ToWorkspace  VariableName=URO_SP1  SampleTime=-1
  Tzew : Step  Time=t0  Before=Tzew0  After=Tzew0+dTzew  SampleTime=0
  Tzew1 : Step  Time=t0  Before=Tzew0  After=Tzew0+dTzew  SampleTime=0
  Tzew2 : Step  Time=t0  Before=Tzew0  After=Tzew0+dTzew  SampleTime=0
  Wartosc zadana1 : Step  Time=t0  Before=Tp0  After=Tp0+dTp  SampleTime=0
  Wartosc zadana2 : Step  Time=t0  Before=Tp0  After=Tp0+dTp  SampleTime=0
  Wartosc zadana3 : Step  Time=t0  Before=Tp0  After=Tp0+dTp  SampleTime=0
  e1 : Scope
  e2 : Scope
  e3 : Scope
  u1 : Scope
  u2 : Scope
  u3 : Scope
  wires:
  Gain12/1 -> Add14/1
  Gain11/1 -> Integrator7/1
  Integrator6/1 -> Add16/1, To Workspace12/1, Sum3/2, Scope6/1, Add13/1  "Temperatura poddasza - obiekt"
  Add17/1 -> Gain14/1
  Gain4/1 -> Add5/3
  Add5/1 -> Gain1/1
  Gain14/1 -> Add11/3
  Gain/1 -> Integrator/1
  Tzew2/1 -> Add17/1, Add13/2
  Add/1 -> Gain2/1
  Add15/1 -> Integrator8/1
  Add8/1 -> Gain8/1
  Add10/1 -> Gain6/1
  PID Controller/1 -> To Workspace5/1, Add5/2, u3/1
  Add12/1 -> Integrator5/1
  Gain6/1 -> Integrator3/1
  Add7/1 -> Integrator4/1
  Add2/1 -> Gain3/1
  Gain3/1 -> Add5/1, Add1/2
  Add9/1 -> Gain9/1
  PID Controller2/1 -> To Workspace14/1, Add11/2, u2/1
  Add11/1 -> Gain11/1
  Gain13/1 -> Add11/1, Add14/2
  Tzew/1 -> Add3/1, Add/2
  Integrator8/1 -> Display3/1
  Gain1/1 -> Integrator1/1
  Add16/1 -> Gain13/1
  Integrator7/1 -> Add17/2, To Workspace13/1, Add16/2, Scope5/1  "Twew(t)"
  Add13/1 -> Gain12/1
  Integrator/1 -> Add2/1, To Workspace/1, Sum1/2, Scope2/1, Add/1  "Temperatura poddasza - obiekt"
  Gain9/1 -> Add10/3
  Integrator5/1 -> Display2/1
  Wartosc zadana3/1 -> To Workspace15/1, Sum3/1
  Gain5/1 -> Integrator2/1
  Wartosc zadana1/1 -> To Workspace7/1, Sum1/1
  Tzew1/1 -> Add9/1, Add4/2
  Add14/1 -> Gain10/1
  Integrator4/1 -> Display1/1
  Wartosc zadana2/1 -> To Workspace9/1, Sum2/1
  Integrator3/1 -> Add9/2, To Workspace4/1, Add8/2, Scope3/1  "Twew(t)"
  Add6/1 -> Gain5/1
  Add3/1 -> Gain4/1
  Gain2/1 -> Add1/1
  Add1/1 -> Gain/1
  Sum2/1 -> e2/1, PID Controller1/1, To Workspace10/1, Add7/2, Add7/1
  PID Controller1/1 -> To Workspace6/1, Add10/2, u1/1
  Sum1/1 -> e1/1, PID Controller/1, To Workspace8/1, Add12/2, Add12/1
  Gain7/1 -> Add6/1
  Gain8/1 -> Add10/1, Add6/2
  Integrator1/1 -> Add3/2, To Workspace1/1, Add2/2, Scope1/1  "Twew(t)"
  Sum3/1 -> e3/1, PID Controller2/1, To Workspace11/1, Add15/2, Add15/1
  Gain10/1 -> Integrator6/1
  Integrator2/1 -> Add8/1, To Workspace3/1, Sum2/2, Scope4/1, Add4/1  "Temperatura poddasza - obiekt"
  Add4/1 -> Gain7/1
